simulink model "MatchedFilterFFT_Transpose"  (R2021a)
settings: Solver=FixedStepDiscrete  StartTime=0.0  StopTime=inf  RelTol=1e-3
InitFcn:
  | FFT2D_matrix_init
values from neighbouring files (symbols this model uses):
  columnWindowFun = taylorwin(nCols,10,-40)    [FFT2D_matrix_init.m]
  DTsig_in = numerictype(1,20,18)    [FFT2D_matrix_init.m]
  DTWindowFun = numerictype(1,16+4,13+4)    [FFT2D_matrix_init.m]
  nCols = 64    [FFT2D_matrix_init.m]
  nRows = 256    [FFT2D_matrix_init.m]
  radarDataCube = createRadarDataCubeMod(     txSignalFullPeriod,antennaElement,Fs,Fc,      targetPos, targetVel, targetRCS,      RngMax, RxActiveTime, RngGate,      CPILength, NumCPI, CPILength*pulsePeriod)    [FFT2D_matrix_init.m]
libraries: hdlsllib x35, simulink x13, hwlogicconnlib x2, dsphdlfiltering x1, dsphdlxfrm x1, dspsrcs4 x1
(part 2 of 2)

== system MatchedFilterFFT_Transpose/HDL_IP/DDRReadWriteController/TransposeMatrix/TotalMatrixSamples ==
  In1 : Inport
  Data Type Conversion : DataTypeConversion  OutDataTypeStr=uint32
  Product : Product  OutDataTypeStr=uint32
  Selector : Selector  InputPortWidth=2  IndexOptions=Index vector (dialog)  Indices=1  OutputSizes=1
  Selector1 : Selector  InputPortWidth=2  IndexOptions=Index vector (dialog)  Indices=2  OutputSizes=1
  Out1 : Outport
  wires:
  In1/1 -> Selector/1, Selector1/1
  Product/1 -> Data Type Conversion/1
  Selector1/1 -> Product/2
  Selector/1 -> Product/1
  Data Type Conversion/1 -> Out1/1

== system MatchedFilterFFT_Transpose/HDL_IP/DDRReadWriteController/TransposeMatrix/WriteToDDR4 ==
  DataIn : Inport
  ValidIn : Inport  Port=2
  WrCmd_s2m_in : Inport  Port=3
  N1_N2 : Inport  Port=4
  Bus Selector : BusSelector  OutputSignals=wr_ready,wr_complete
  DataWrLogic : Subsystem
  Selector : Selector  InputPortWidth=2  IndexOptions=Index vector (dialog)  Indices=1  OutputSizes=1
  Selector1 : Selector  InputPortWidth=2  IndexOptions=Index vector (dialog)  Indices=2  OutputSizes=1
  WrCmd_m2s : hwlogicconnlib/SoC Bus Creator  Protocol=Random access write  ctrltype=Valid
      settings: SourceProductBaseCode=HW
  WrCmd_s2m_out : Outport
  WrData_s2m_out : Outport  Port=2
  matrix_wr_done : Outport  Port=3
  wr_full : Outport  Port=4
  wires:
  DataWrLogic/4(wr_valid) -> WrCmd_m2s/3  "WrValid"
  DataWrLogic/3(wr_len) -> WrCmd_m2s/2  "WrLen"
  ValidIn/1 -> DataWrLogic/2(ValidIn)
  DataWrLogic/2(wr_addr) -> WrCmd_m2s/1  "WrAddr"
  DataWrLogic/1(data) -> WrData_s2m_out/1  "WrData_s2m"
  Bus Selector/2 -> DataWrLogic/4(wr_complete)  "<wr_complete>"
  DataIn/1 -> DataWrLogic/1(DataIn)
  WrCmd_m2s/1 -> WrCmd_s2m_out/1
  Bus Selector/1 -> DataWrLogic/3(wr_Ready)  "<wr_ready>"
  WrCmd_s2m_in/1 -> Bus Selector/1
  DataWrLogic/5(matrix_wr_done) -> matrix_wr_done/1
  DataWrLogic/6(AlmostFull) -> wr_full/1
  N1_N2/1 -> Selector/1, Selector1/1
  Selector/1 -> DataWrLogic/5(N1)
  Selector1/1 -> DataWrLogic/6(N2)

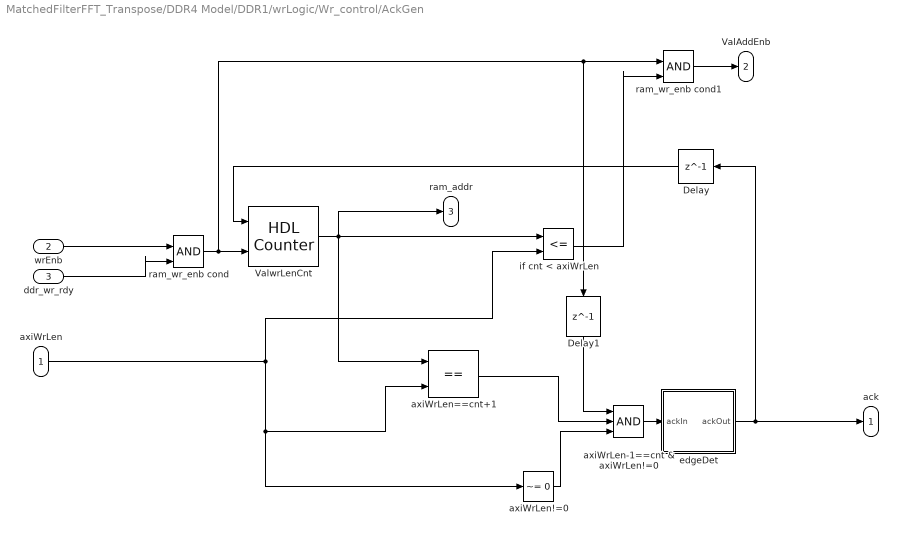
== system MatchedFilterFFT_Transpose/DDR4 Model/DDR1/wrLogic/Wr_control/AckGen ==
  axiWrLen : Inport
  wrEnb : Inport  Port=2
  ddr_wr_rdy : Inport  Port=3
  Delay : Delay  DelayLength=1
  Delay1 : Delay  DelayLength=1
  ValwrLenCnt : hdlsllib/Sources/HDL Counter  CountType=Free running  CountInit=0  CountStep=1  CountMax=DDR3_DEPTH  CountFromType=Initial value  CountFrom=0  CountResetPort=on  CountLoadPort=off  CountEnbPort=on  CountDirPort=off  CountHitOutputPort=off  CountDataType=Unsigned  CountWordLen=32  CountFracLen=0  CountSampTime=1
  axiWrLen!=0 : simulink/Logic and Bit Operations/Compare To Constant  relop=~=  const=0  OutDataTypeStr=boolean
  "axiWrLen-1==cnt & axiWrLen!=0 " : Logic  Inputs=3  IconShape=distinctive  AllPortsSameDT=off  OutDataTypeStr=boolean
  axiWrLen==cnt+1 : RelationalOperator  Operator===  OutDataTypeStr=boolean  RndMeth=Nearest
  edgeDet : Subsystem
  if cnt < axiWrLen : RelationalOperator  Operator=<=  OutDataTypeStr=boolean  RndMeth=Nearest
  ram_wr_enb cond : Logic  IconShape=distinctive  AllPortsSameDT=off  OutDataTypeStr=boolean
  ram_wr_enb cond1 : Logic  IconShape=distinctive  AllPortsSameDT=off  OutDataTypeStr=boolean
  ack : Outport  VectorParamsAs1DForOutWhenUnconnected=off
  ValAddEnb : Outport  Port=2  VectorParamsAs1DForOutWhenUnconnected=off
  ram_addr : Outport  Port=3  VectorParamsAs1DForOutWhenUnconnected=off
  wires:
  Delay1/1 -> "axiWrLen-1==cnt & axiWrLen!=0 "/1
  Delay/1 -> ValwrLenCnt/1
  ram_wr_enb cond1/1 -> ValAddEnb/1
  ram_wr_enb cond/1 -> ValwrLenCnt/2, Delay1/1, ram_wr_enb cond1/1
  ddr_wr_rdy/1 -> ram_wr_enb cond/2
  ValwrLenCnt/1 -> ram_addr/1, if cnt < axiWrLen/1, axiWrLen==cnt+1/1
  axiWrLen/1 -> if cnt < axiWrLen/2, axiWrLen!=0/1, axiWrLen==cnt+1/2
  if cnt < axiWrLen/1 -> ram_wr_enb cond1/2
  wrEnb/1 -> ram_wr_enb cond/1
  axiWrLen!=0/1 -> "axiWrLen-1==cnt & axiWrLen!=0 "/3
  axiWrLen==cnt+1/1 -> "axiWrLen-1==cnt & axiWrLen!=0 "/2
  edgeDet/1(ackOut) -> Delay/1, ack/1
  "axiWrLen-1==cnt & axiWrLen!=0 "/1 -> edgeDet/1(ackIn)

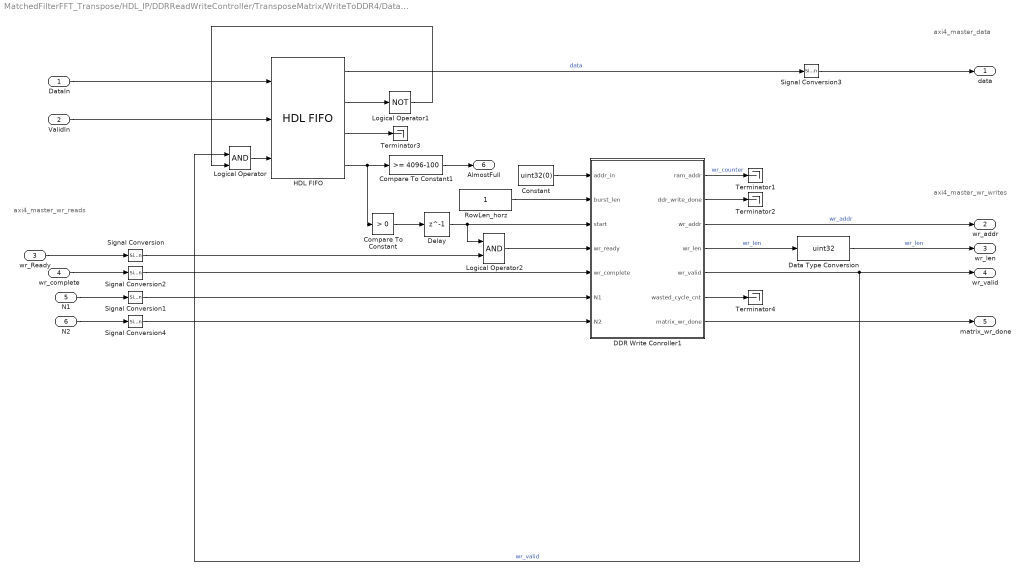
== system MatchedFilterFFT_Transpose/HDL_IP/DDRReadWriteController/TransposeMatrix/WriteToDDR4/DataWrLogic ==
  note: axi4_master_wr_reads
  note: axi4_master_wr_writes
  note: axi4_master_data
  DataIn : Inport
  ValidIn : Inport  Port=2
  wr_Ready : Inport  Port=3
  wr_complete : Inport  Port=4
  N1 : Inport  Port=5
  N2 : Inport  Port=6
  Compare To Constant : simulink/Logic and Bit Operations/Compare To Constant  relop=>  const=0  OutDataTypeStr=boolean
  Compare To Constant1 : simulink/Logic and Bit Operations/Compare To Constant  relop=>=  const=4096-100  OutDataTypeStr=boolean
  Constant : Constant  Value=uint32(0)  SampleTime=-1
  DDR Write Conroller1 : MATLAB Function  TreatAsAtomicUnit=on
  Data Type Conversion : DataTypeConversion  OutDataTypeStr=uint32
  Delay : Delay  DelayLength=1
  HDL FIFO : hdlsllib/HDL RAMs/HDL FIFO  fifo_size=4096  mode=FWFT  ratio=1  push_msg=Warning  pop_msg=Warning  show_empty=on  show_full=on  show_num=on  LabelModeActiveChoice_Mode=FWFT
      settings: SourceProductBaseCode=SL
  Logical Operator : Logic  IconShape=distinctive  AllPortsSameDT=off  OutDataTypeStr=boolean
  Logical Operator1 : Logic  Operator=NOT  IconShape=distinctive  AllPortsSameDT=off  OutDataTypeStr=boolean
  Logical Operator2 : Logic  IconShape=distinctive  AllPortsSameDT=off  OutDataTypeStr=boolean
  RowLen_horz : Constant  OutDataTypeStr=uint32  SampleTime=-1
  Signal Conversion{,1..4} (5 alike) : SignalConversion  OverrideOpt=off
  Terminator{1..4} (4 alike) : Terminator
  data : Outport
  wr_addr : Outport  Port=2
  wr_len : Outport  Port=3
  wr_valid : Outport  Port=4
  matrix_wr_done : Outport  Port=5
  AlmostFull : Outport  Port=6
  wires:
  ValidIn/1 -> HDL FIFO/2
  Data Type Conversion/1 -> wr_len/1  "wr_len"
  DataIn/1 -> HDL FIFO/1
  HDL FIFO/1 -> Signal Conversion3/1  "data"
  wr_complete/1 -> Signal Conversion2/1
  wr_Ready/1 -> Signal Conversion/1
  HDL FIFO/2 -> Logical Operator1/1
  Logical Operator/1 -> HDL FIFO/3
  Signal Conversion/1 -> Logical Operator2/2
  Logical Operator2/1 -> DDR Write Conroller1/4(wr_ready)
  Logical Operator1/1 -> Logical Operator/2
  Compare To Constant/1 -> Delay/1
  Signal Conversion2/1 -> DDR Write Conroller1/5(wr_complete)
  RowLen_horz/1 -> DDR Write Conroller1/2(burst_len)
  DDR Write Conroller1/5(wr_valid) -> Logical Operator/1, wr_valid/1  "wr_valid"
  Signal Conversion3/1 -> data/1
  HDL FIFO/3 -> Terminator3/1
  Delay/1 -> Logical Operator2/1, DDR Write Conroller1/3(start)
  Constant/1 -> DDR Write Conroller1/1(addr_in)
  HDL FIFO/4 -> Compare To Constant/1, Compare To Constant1/1
  Compare To Constant1/1 -> AlmostFull/1
  N2/1 -> Signal Conversion4/1
  N1/1 -> Signal Conversion1/1
  Signal Conversion1/1 -> DDR Write Conroller1/6(N1)
  Signal Conversion4/1 -> DDR Write Conroller1/7(N2)
  DDR Write Conroller1/3(wr_addr) -> wr_addr/1  "wr_addr"
  DDR Write Conroller1/4(wr_len) -> Data Type Conversion/1  "wr_len"
  DDR Write Conroller1/7(matrix_wr_done) -> matrix_wr_done/1
  DDR Write Conroller1/6(wasted_cycle_cnt) -> Terminator4/1
  DDR Write Conroller1/2(ddr_write_done) -> Terminator2/1
  DDR Write Conroller1/1(ram_addr) -> Terminator1/1  "wr_counter"

== system MatchedFilterFFT_Transpose/DDR4 Model/DDR1/wrLogic/Wr_control/AckGen/edgeDet ==
  ackIn : Inport
  " ackIn==1" : simulink/Logic and Bit Operations/Compare To Constant  relop===  const=1  OutDataTypeStr=boolean
  ackIn Posedge Detect : Logic  IconShape=distinctive  AllPortsSameDT=off  OutDataTypeStr=boolean
  ackIn_d1 : Delay  DelayLength=1
  ackIn_d1==0 : simulink/Logic and Bit Operations/Compare To Constant  relop===  const=0  OutDataTypeStr=boolean
  ackOut : Outport  VectorParamsAs1DForOutWhenUnconnected=off
  wires:
  ackIn/1 -> ackIn_d1/1, " ackIn==1"/1
  ackIn_d1/1 -> ackIn_d1==0/1
  ackIn Posedge Detect/1 -> ackOut/1
  ackIn_d1==0/1 -> ackIn Posedge Detect/1
  " ackIn==1"/1 -> ackIn Posedge Detect/2

== matlab function MatchedFilterFFT_Transpose/DDR4 Model/DDR1/rdLogic/rd_control ==
  data: axi_rd_add input; axi_rd_len input; axi_rd_val input; axi_rd_ready input; ram_rd_addr output; ram_rd_val output boolean; toggle parameter; WR_RD_DATAWIDTH parameter; rdDone output
function [ram_rd_addr, ram_rd_val, rdDone] = rd_add_gen(axi_rd_add,axi_rd_len, axi_rd_val,axi_rd_ready,toggle, WR_RD_DATAWIDTH)

%%%%%%%%%%%%%%%%%%%%%%%%%%%%%%%%%%%%%%%%%%%%%%%%%%%%%%
%%%Reg declaration
%RAM address generation counter
persistent ram_rd_cnt;

RD_BYTE_STRIDE = uint32(WR_RD_DATAWIDTH/8);
rdDone = false;

if(isempty(ram_rd_cnt))
    ram_rd_cnt = fi(0,0,32,0);%uint32(0);
end

%read response ack
persistent reg_rd_ack;

if(isempty(reg_rd_ack))
    reg_rd_ack = false;
end

%read status
persistent rd_progress;

if(isempty(rd_progress))
    rd_progress = false;
end

%read addr valid flag 
persistent rd_addr_val;

if(isempty(rd_addr_val))
    rd_addr_val = false;
end

%read addr valid flag 
persistent rd_addr_val_toggle;

if(isempty(rd_addr_val_toggle))
    rd_addr_val_toggle = false;
end

%start address and length of read burst latch
persistent start_addr;
if(isempty(start_addr))
    start_addr = fi(0,0,32,0);
end

persistent leng_latch;
if(isempty(leng_latch))
    leng_latch = fi(1,0,32,0);
end

%%%%%%%%%%%%%%%%%%%%%%%%%%%%%%%%%%%%%%%%%%%%%%%
%output
ram_rd_addr = (ram_rd_cnt);
ram_rd_val = (rd_addr_val);
%%%%%%%%%%%%%%%%%%%%%%%%%%%%%%%%%%%%%%%%%%%%%%%
if((reg_rd_ack == true)&&(axi_rd_ready == true))
    ram_rd_cnt = fi(start_addr,0,32,0);%uint32(start_addr );
    rd_addr_val = true;
elseif((rd_progress == true)&&(axi_rd_ready == true))
    
    if(rd_addr_val_toggle == true)
       ram_rd_cnt = fi(ram_rd_cnt + 1,0,32,0);%uint32(ram_rd_cnt + 1);
       rd_addr_val = true;
    else
       rd_addr_val = false;
   
    end
    if(toggle)
       rd_addr_val_toggle = ~(rd_addr_val_toggle);
    else
       rd_addr_val_toggle = true;
    end
    
    TargetVal = (int32(leng_latch-1) - 1);
    if int32(ram_rd_cnt) == TargetVal
            rdDone = true;
    end
    
elseif((rd_progress == false))  
    ram_rd_cnt = fi(0,0,32,0);%uint32(0) ;
    rd_addr_val = false;
else
    rd_addr_val = false;
end


%read progress flag
if((reg_rd_ack)&&(fi(ram_rd_cnt-start_addr,0,32,0)<fi(leng_latch-1,0,32,0)))
    rd_progress = true;
elseif(fi(ram_rd_cnt-start_addr,0,32,0)==fi(leng_latch-1,0,32,0))
    rd_progress = false;
    rdDone = true; 
end


%start address , length of burst latching
if(axi_rd_val)
    leng_latch(:) = axi_rd_len;
    start_addr(:) = axi_rd_add/RD_BYTE_STRIDE;
    reg_rd_ack = true;
elseif rd_progress == false
    rdDone = true; 
    reg_rd_ack = false;
else
    reg_rd_ack = false;
end

== matlab function MatchedFilterFFT_Transpose/DDR4 Model/DDR1/wrLogic/Wr_control/MATLAB Function ==
  data: axi_wr_en input; wr_leng output; axi_wr_length input; wr_ack input; wr_done_o output
function [wr_leng,wr_done_o]= addr_latch(axi_wr_en,axi_wr_length,wr_ack)
%#codegen

persistent axi_wr_en_d1 write_done init_count fifo_counter;
if(isempty(axi_wr_en_d1))
axi_wr_en_d1 = false;
write_done = true;
init_count = false;
fifo_counter  = uint32(0);
end

persistent reg_len;
if(isempty(reg_len))
    reg_len = fi(0,0,32,0);%uint32(0);
end


persistent reg_len_d1;
if(isempty(reg_len_d1))
    reg_len_d1 = fi(0,0,32,0);%uint32(0);
end

reg_len_d1 = reg_len;
wr_leng = reg_len;

if((axi_wr_en==true)&&(axi_wr_en_d1==false)&&(reg_len_d1==0)) 
  reg_len= fi(axi_wr_length,0,32,0);%axi_wr_length;
  init_count = true;
  write_done = false;  % not ready to receive new data, processing current frames
  fifo_counter = uint32(0);
elseif(wr_ack)
  reg_len= fi(0,0,32,0);%uint32(0);  
  write_done = true;  % ready to receive new data
end

% if init_count
%     if fifo_counter >= axi_wr_length
%         init_count = false;
%     else
%         fifo_counter = fifo_counter + 1;
%         write_done = true;
%     end
%    
% end

% if init_count
%     % count to axi_wr_length
%     % while less than axi_wr_length, set write_done = true
%     % after we reach count, set init_count = false
%     if fifo_counter >= axi_wr_length
%         init_count = false;   
%         wr_done_o = false;
%     else
%         fifo_counter = fifo_counter + 1;
%         wr_done_o = true;
%     end
% end
 wr_done_o = write_done;

axi_wr_en_d1 = axi_wr_en;

== matlab function MatchedFilterFFT_Transpose/DDR4 Model/DDR1/wr_queue/MATLAB Function ==
  data: valid_in input; pop_in input; pop_ctrl output; wr_len input
function pop_ctrl = fcn(valid_in, pop_in, wr_len)

persistent state_ctrl wr_len_reg counter;
if isempty(state_ctrl)
    state_ctrl = fi(0,0,4,0);
    counter = uint32(0);
    wr_len_reg = uint32(0);
end
STATE_IDLE = fi(0,0,4,0);
STATE_PROCESSING  = cast(1,'like',STATE_IDLE);
pop_ctrl = false;
switch(state_ctrl)
    case(STATE_IDLE)
        if valid_in
            wr_len_reg(:) = wr_len;
        end
        if pop_in == true
            pop_ctrl = true;
            state_ctrl(:) = STATE_PROCESSING;
            counter(:) = 1;
        end
    case(STATE_PROCESSING)
        
        
        if counter >= wr_len_reg
            pop_ctrl = false;
            state_ctrl(:) = STATE_IDLE;
        else
            pop_ctrl = true;
            counter(:) = counter+ 1;
        end
end

end

== matlab function MatchedFilterFFT_Transpose/ReadMatrixData ==
  data: sigOut output; valid_out output; MatrixInput parameter; row_counter_o output; col_counter_o output; ValidGap parameter; ready input
function [sigOut,valid_out,row_counter_o,col_counter_o] = fcn(MatrixInput,ValidGap, ready)
    persistent row_counter col_counter stop_write;
%     ValidGap = 10;
    if isempty(row_counter)
        row_counter = uint32(1);
        col_counter = uint32(1);
        stop_write = false;
      
    end
    [n_rows,m_cols] = size(MatrixInput);
    max_row_count = n_rows + ValidGap;

    %% Read value from matrix
    if row_counter <= n_rows && ~stop_write
        sigOut = MatrixInput(row_counter,col_counter);
        valid_out = true;
    else
        sigOut = 0; % insert valid gap 
        valid_out = false;
    end
    
    row_counter_o = row_counter;
    col_counter_o = col_counter;
    
    %% Update counters
    if ready
        if row_counter < max_row_count 
            row_counter(:) = row_counter + 1; 
        else
            row_counter(:) = 1;
            if col_counter < m_cols
                col_counter(:) = col_counter + 1; % next column
            else
                col_counter(:) = 1; % reset to beginning of matrix
                stop_write = false; % set to false to stop indefinite reads
            end
        end
    else
        valid_out = false;
    end

end

== matlab function MatchedFilterFFT_Transpose/HDL_IP/DDRReadWriteController/TransposeMatrix/WriteToDDR4/DataWrLogic/DDR Write Conroller1 ==
  data: addr_in input; ram_addr output; ddr_write_done output; burst_len input; start input boolean; wr_ready input; wr_addr output; wr_len output; wr_valid output; wr_complete input; wasted_cycle_cnt output; matrix_wr_done output; N1 input uint32; N2 input uint32
function [ram_addr, ddr_write_done, wr_addr, wr_len, wr_valid, wasted_cycle_cnt, matrix_wr_done] = ...
    hdlcoder_external_memory_write_ctrl_custom(addr_in,burst_len, start, wr_ready, wr_complete,N1, N2)
%% hdlcoder_external_memory_write_ctrl_custom
%
% % State-machine behavior for writing to DDR4

%   Copyright 2017 The MathWorks, Inc.

% create persistent variables (registers)
persistent wstate burst_stop burst_count wasted_cycle_count % Diagnostics
persistent addr_value addr_offset_add % address and offset
persistent N1_reg N2_reg % Matrix dimensions
if(isempty(wstate))
    wstate      = fi(0, 0, 4, 0);
    burst_stop  = uint32(0);
    burst_count = uint32(0);
    wasted_cycle_count = uint32(0);    
    addr_value = uint32(0);
    addr_offset_add = uint32(0);
    N1_reg = uint32(0);
    N2_reg = uint32(0);
end
wasted_cycle_cnt = cast(0,'like',wasted_cycle_count);

% state machine encoding
IDLE              = fi(0, 0, 4, 0);
WRITE_BURST_START = fi(1, 0, 4, 0);
DATA_COUNT        = fi(2, 0, 4, 0);
ACK_WAIT          = fi(3, 0, 4, 0);

DATA_BYTE_SIZE = uint32(8); % we are using a 64-bit data bus for this


% state machine logic
switch (wstate)
    case IDLE
        % output to AXI4 Master
        wr_addr  = uint32(0); % 4-byte address
        wr_len   = uint32(0);
        wr_valid = false;
        
        % output to DUT logic
        ram_addr = uint32(0);
        ddr_write_done = true;
        matrix_wr_done = false;
        
        % state variables
        burst_stop  = uint32(burst_len);
        burst_count = uint32(0);
        
        if start
            wstate(:) = WRITE_BURST_START;
            N1_reg(:) = N1; % Update matrix dimensions and use this for the remainder of the burst
            N2_reg(:) = N2;
        else
            wstate(:) = IDLE;
        end
        
        
    case WRITE_BURST_START
        % output to AXI4 Master
        wr_addr  = uint32((addr_value+addr_offset_add)*DATA_BYTE_SIZE); % convert to bytes
        wr_len   = uint32(burst_stop);
        wr_valid = false;
        
        % output to DUT logic
        ram_addr = uint32(burst_count);
        ddr_write_done = false;
        matrix_wr_done = false;    
        
        if wr_ready
            wstate(:) = DATA_COUNT;
        else
            wstate(:) = WRITE_BURST_START;
            wasted_cycle_count = uint32(wasted_cycle_count+1);
        end
        
        
    case DATA_COUNT
        % output to AXI4 Master
        wr_addr  = uint32((addr_value+addr_offset_add)*DATA_BYTE_SIZE); % convert to bytes
        wr_len   = uint32(burst_stop);
        wr_valid = true;
        
        % state variables
        burst_count = uint32(burst_count + 1);
        
        % output to DUT logic
        ram_addr = uint32(burst_count);
        ddr_write_done = false;
        matrix_wr_done = false;
        
        if ( burst_count == burst_stop )
            wstate(:) = ACK_WAIT;            
        else
            if ( wr_ready )
                wstate(:) = DATA_COUNT;
            else
                wstate(:) = WRITE_BURST_START;
            end
        end
        
        
    case ACK_WAIT
        % output to AXI4 Master
        wr_addr  = uint32(0);
        wr_len   = uint32(0);
        wr_valid = false;
        
        % output to DUT logic
        ram_addr = uint32(0);
        ddr_write_done = false;
        matrix_wr_done = false;
        
        if wr_complete
            wstate(:) = IDLE;
                   
            if addr_value < (N2_reg*(N1_reg-1)) % Address stride will be 0:N2_reg:N2_reg*(N1_reg-1)
                % Small example (N1_reg=4,N2_reg=5):
                %   0 1 2 3 4
                %   5 6 7 8 9
                %   10 11... etc 
                addr_value(:) = addr_value + (N2_reg);
            else
                
                if addr_offset_add < (N2_reg-1)  % Will add an offset value to above addresses for each column
                                             % Using the small N1_reg=4 and
                                             % N2_reg=5 example...
                                             % 0,1,2,3,4 are used to offset
                                             % the above addreses
                                             % horizontally
                    addr_offset_add(:) = addr_offset_add + 1;
                else
                    addr_offset_add(:) = 0;
                    matrix_wr_done = true; 
                end    
                
                addr_value(:) = 0 ; % perform reset on address
            end
        else
            wstate(:) = ACK_WAIT;
        end
        
    otherwise
        % output to AXI4 Master
        wr_addr = uint32(0);
        wr_len = uint32(0);
        wr_valid = false;
        matrix_wr_done = false;
        
        % output to DUT logic
        ram_addr = uint32(0);
        ddr_write_done = false;
        
        wstate(:) = IDLE;
        
end
    
% For AXI4 MM Diagonstics
wasted_cycle_cnt(:) = wasted_cycle_count;

end

% LocalWords:  AXI

== matlab function MatchedFilterFFT_Transpose/HDL_IP/DDRReadWriteController/TransposeMatrix/ReadFromDDR4/DDR Read Conroller ==
  data: valid_out output; count_out output; ddr_read_done output; burst_len input; start input boolean; rd_aready input; rd_dvalid input; rd_addr output; rd_len output; rd_avalid output; ToggleTLAST output; debug_state output
function [valid_out, count_out, ddr_read_done, rd_addr, rd_len, rd_avalid,ToggleTLAST,debug_state] = ...
    hdlcoder_external_memory_read_ctrl_custom(burst_len, start, rd_aready, rd_dvalid)
%% hdlcoder_external_memory_read_ctrl_custom
%
% % State-machine behavior for reading DDR4

%   Copyright 2017 The MathWorks, Inc.

% create persistent variables (registers)
persistent rstate burst_stop burst_count
if isempty(rstate)
    rstate      = fi(0, 0, 4, 0);
    burst_stop  = uint32(0);
    burst_count = uint32(0);
    debug_state = cast(0,'like',rstate);
end

% state Memory Encoding
IDLE               = fi(0, 0, 4, 0);
READ_BURST_START   = fi(1, 0, 4, 0);
READ_BURST_REQUEST = fi(2, 0, 4, 0);
DATA_COUNT         = fi(3, 0, 4, 0);

ToggleTLAST = false;

% state machine logic
switch (rstate)
    case IDLE
        % output to AXI4 Master
        rd_addr   = uint32(0);
        rd_len    = uint32(0);
        rd_avalid = false;
        
        % output to DUT logic
        valid_out = false;
        count_out = uint32(0);
        ddr_read_done = true;
        
        % State vars
        burst_stop  = uint32(burst_len);
        burst_count = uint32(0);
        
        if start
            rstate(:) = READ_BURST_START;
        else
            rstate(:) = IDLE;
        end
        
    case READ_BURST_START
        % Daren Notes: the two pieces of information below is a read request
        %
        % rd_addr: Starting address for the read transaction that is sampled at 
        %          the first cycle of the transaction.
        % rd_len: The number of data values that you want to read, 
        %         sampled at the first cycle of the transaction.
        %
        % We only move to READ_BURST_REQUST if rd_aready is HIGH to confirm
        % DDR is ready for a readback request
        
        % output to AXI4 Master
        rd_addr   = uint32(0);  
        rd_len    = uint32(burst_stop);
        rd_avalid = false;
        
        % output to DUT logic
        valid_out = false;
        count_out = uint32(0);
        ddr_read_done = false;
        
        if rd_aready
            rstate(:) = READ_BURST_REQUEST;
        else
            rstate(:) = READ_BURST_START;
        end
        
    case READ_BURST_REQUEST
        % Daren Notes: read request
        %
        % rd_avalid: Control signal that specifies whether the read request is valid.
        %
        %
        
        % output to AXI4 Master
        rd_addr   = uint32(0);
        rd_len    = uint32(burst_stop);
        rd_avalid = true;
        
        % output to DUT logic
        valid_out = false;
        count_out = uint32(0);
        ddr_read_done = false;
        
        rstate(:) = DATA_COUNT;
        
    case DATA_COUNT
        % output to AXI4 Master
        rd_addr   = uint32(0);
        rd_len    = uint32(burst_stop);
        rd_avalid = false;
        
        % output to DUT logic
        valid_out = rd_dvalid;
        count_out = uint32(burst_count);
        ddr_read_done = false;
        
        % State vars
        if ( rd_dvalid )
            burst_count = uint32(burst_count + 1);
        end
        
        if ( burst_count == burst_stop )
            rstate(:) = IDLE;
            if rd_dvalid
                ToggleTLAST = true;
            end
        else
            rstate(:) = DATA_COUNT;
        end
        
    otherwise
        % output to AXI4 Master
        rd_addr   = uint32(0);
        rd_len    = uint32(0);
        rd_avalid = false;
        
        % output to DUT logic
        valid_out = false;
        count_out = uint32(0);
        ddr_read_done = false;
        
        rstate(:) = IDLE;
end

debug_state(:) = rstate;

end

% LocalWords:  AXI

== matlab function MatchedFilterFFT_Transpose/DDR4 Model/DDR1/load_init_data ==
  data: load_done output; ram_wr_data output; axi_wr_data input; axi_wr_add input; axi_wr_val input; ram_wr_add output; ram_wr_enb output boolean; INIT_ADDR parameter; DDR3_DEPTH parameter; INIT_DDR3 parameter; INIT_DATA parameter
function [load_done,ram_wr_data,ram_wr_add,ram_wr_enb] = load_init(axi_wr_data,axi_wr_add,axi_wr_val, INIT_ADDR, DDR3_DEPTH, INIT_DDR3,INIT_DATA)

%%%%%%%%%%%%%%%%%%%%%%%%%%%%%%%%%%%%%%%%%%%%%%%%%%%%%%
% Create persistent variables (registers)
persistent reg_ram_wr_add;
if(isempty(reg_ram_wr_add))
    reg_ram_wr_add = fi(0,0,32,0);
end

ram_wr_data = cast(0,'like',axi_wr_data);

persistent reg_ram_wr_data;
if(isempty(reg_ram_wr_data))
    reg_ram_wr_data =cast(0,'like',axi_wr_data);% fi(0,1,ddrWidth,0);
end

persistent reg_ram_wr_data_d1;
if(isempty(reg_ram_wr_data_d1))
    reg_ram_wr_data_d1 = cast(0,'like',axi_wr_data);%
end


persistent state;
if(isempty(state))
    state = fi(0, 0, 3, 0);
end


persistent reg_ram_wr_enb;
if(isempty(reg_ram_wr_enb))
    reg_ram_wr_enb = false;
end

persistent reg_ram_wr_enb_d1;
if(isempty(reg_ram_wr_enb_d1))
    reg_ram_wr_enb_d1 = false;
end

persistent reg_init_data;
if(isempty(reg_init_data))
    reg_init_data = cast(zeros(1,DDR3_DEPTH),'like',axi_wr_data);% fi(zeros(1,DDR3_DEPTH),1,ddrWidth,0);
end

%%%%%%%%%%%%%%%%%%%%%%%%%%%%%%%%%%%%%%%%%%%%%%%%%%
% State Memory Encoding
INIT_ST    = fi(0, 0, 3, 0);
LOAD_START = fi(1, 0, 3, 0);
LOAD_PROG  = fi(3, 0, 3, 0);
LOAD_DONE  = fi(2, 0, 3, 0);
DATA_ST    = fi(6, 0, 3, 0);


% init phase states
% 1. Every state MUST assign every output value
% 2. Use explicit data type always
switch (state)
    case INIT_ST
       
        reg_ram_wr_add = fi(0,0,32,0);%uint32(0);
        reg_ram_wr_data =  cast(0,'like',axi_wr_data);%fi(0,1,ddrWidth,0);%int32(0);
        reg_ram_wr_enb = false;
        load_done = false;
        
    case LOAD_START
        
        reg_ram_wr_add = fi(INIT_ADDR,0,32,0);
        reg_ram_wr_data =  cast(reg_init_data(1,reg_ram_wr_add+1),'like',axi_wr_data);%fi(reg_init_data(1,reg_ram_wr_add+1),1,ddrWidth,0);%int32(INIT_DATA);
        reg_ram_wr_enb = true;
        load_done = false;
    case LOAD_PROG
        
        
        reg_ram_wr_add = fi(reg_ram_wr_add+1,0,32,0);
        reg_ram_wr_data =  cast(reg_init_data(1,reg_ram_wr_add+1),'like',axi_wr_data);%fi(reg_init_data(1,reg_ram_wr_add+1),1,ddrWidth,0);%int32(INIT_DATA);
        reg_ram_wr_enb = true;
        load_done = false;
    case LOAD_DONE
      
        reg_ram_wr_add = fi(reg_ram_wr_add,0,32,0);
       % reg_ram_wr_data = reg_ram_wr_data;%fi(reg_ram_wr_data,1,ddrWidth,0);
        reg_ram_wr_enb = true;
        load_done = true;
    case DATA_ST    
        %external (AXI ) inputs
        reg_ram_wr_add = fi(axi_wr_add,0,32,0);
        reg_ram_wr_data =  axi_wr_data;%fi(axi_wr_data,1,ddrWidth,0);
        reg_ram_wr_enb = axi_wr_val;
        load_done = true;
    otherwise
        
        reg_ram_wr_add = fi(0,0,32,0);
        reg_ram_wr_data =  cast(0,'like',axi_wr_data);%fi(0,1,ddrWidth,0);
        reg_ram_wr_enb = false;
        load_done = false;
end

ram_wr_add = fi(reg_ram_wr_add,0,32,0);
%ram_wr_data = reg_ram_wr_data;

if(load_done == true)
   ram_wr_data = cast(reg_ram_wr_data_d1,'like',axi_wr_data);%fi(reg_ram_wr_data_d1,1,ddrWidth,0);%reg_ram_wr_data_d1;
else
   ram_wr_data = cast(reg_ram_wr_data_d1,'like',axi_wr_data);%fi(reg_ram_wr_data_d1,1,ddrWidth,0);%reg_ram_wr_data;   
end


if(load_done == true)
   ram_wr_enb = reg_ram_wr_enb_d1;
else
   ram_wr_enb = reg_ram_wr_enb;   
end


if(load_done == false)
   reg_init_data = cast(INIT_DATA,'like',axi_wr_data);%fi(INIT_DATA,1,ddrWidth,0);%reg_ram_wr_data;   
end

reg_ram_wr_enb_d1 = reg_ram_wr_enb;
reg_ram_wr_data_d1 = reg_ram_wr_data;%fi(reg_ram_wr_data,1,ddrWidth,0);%int32(reg_ram_wr_data);
% Next State Logic
switch (state)
    case INIT_ST
        
        if ( INIT_DDR3 == true)
            nextState = LOAD_START;
        else
            nextState = DATA_ST;
        end
    case LOAD_START
            nextState = LOAD_PROG;
    case LOAD_PROG
        if(fi(ram_wr_add,0,32,0)==fi(DDR3_DEPTH-1,0,32,0))
            nextState = LOAD_DONE;
        else
            nextState = LOAD_PROG;
        end
    case LOAD_DONE
            nextState = DATA_ST;
    case DATA_ST
            nextState = DATA_ST; 
    otherwise
        nextState = INIT_ST;
end

state = nextState;

end

== matlab function MatchedFilterFFT_Transpose/DDR4 Model/DDR1/rdLogic/axim_rd_aready_behavior ==
  data: rdDonePulse input; rd_rdy output
function rd_rdy = aready(rdDonePulse)

persistent rdy_state delay_count
if isempty(rdy_state)
    rdy_state = uint32(0);
    delay_count = uint8(0);
end

STATE_IDLE = uint32(0);
STATE_WAIT = uint32(1);
WAIT_TIME = uint16(50);
rd_rdy = false;



switch(rdy_state)
    case(STATE_IDLE)
        if rdDonePulse % if a read just completed, wait a few moments
            rdy_state(:) = STATE_WAIT;            
        else
            rd_rdy = true;
        end
        
    case(STATE_WAIT)
        rd_rdy = false;
        
        if delay_count == WAIT_TIME
            delay_count(:) = 0;
            rdy_state(:) = STATE_IDLE;
        else
            delay_count(:) = delay_count + 1;
        end
    otherwise
        rd_rdy = false;        
end


end
